simulink model "lab4"  (R2017b)
settings: Solver=FixedStepAuto  StartTime=0.0  StopTime=1  FixedStep=0.01  RelTol=1e-3
undefined symbols (not defined in the file): serial
libraries: instrumentlib x3
settings Model: Creator=Студент  LastModifiedBy=Студент

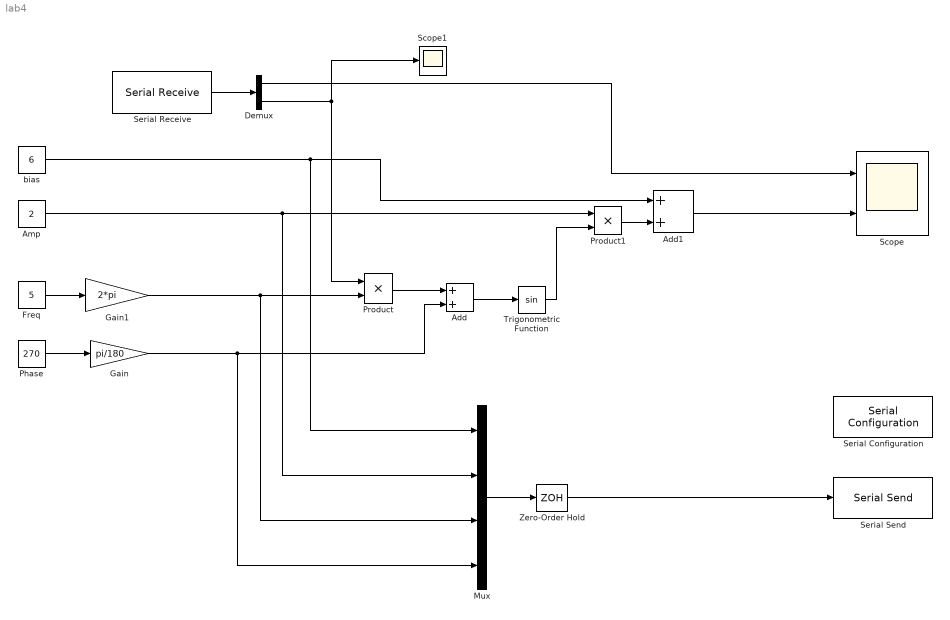
== system lab4 ==
  Add : Sum
  Add1 : Sum
  Amp : Constant  Value=2
  Demux : Demux  Outputs=2
  Freq : Constant  Value=5
  Gain : Gain  Gain=pi/180
  Gain1 : Gain  Gain=2*pi
  Mux : Mux
  Phase : Constant  Value=270
  Product : Product
  Product1 : Product
  Scope : Scope  NumInputPorts=2
  Scope1 : Scope
  Serial Configuration : instrumentlib/Serial Configuration  Priority=-200000  ComPortMenu=COM3  ComPort=COM3  ObjConstructor=serial('COM3');  BaudRate=19200  DataBits=8  Parity=none  StopBits=1  FlowControl=none  Timeout=10  ByteOrder=LittleEndian
  Serial Receive : instrumentlib/Serial Receive  ComPortMenu=COM3  ComPort=COM3  ObjConstructor=serial('COM3');  Terminator=<none>  DataSize="[1  2]"  DataType=double  EnableBlockingMode=on  ActionDataUnavailable=Output last received value  CustomValue=0  SampleTime=0.01
  Serial Send : instrumentlib/Serial Send  ComPortMenu=COM3  ComPort=COM3  ObjConstructor=serial('COM3');  Terminator=<none>  EnableBlockingMode=on
  Trigonometric Function : Trigonometry
  Zero-Order Hold : ZeroOrderHold  SampleTime=-1
  bias : Constant  Value=6  OutDataTypeStr=double
  wires:
  bias/1 -> Mux/1, Add1/1
  Amp/1 -> Mux/2, Product1/1
  Freq/1 -> Gain1/1
  Phase/1 -> Gain/1
  Product/1 -> Add/1
  Add/1 -> Trigonometric Function/1
  Trigonometric Function/1 -> Product1/2
  Product1/1 -> Add1/2
  Add1/1 -> Scope/2
  Zero-Order Hold/1 -> Serial Send/1
  Gain/1 -> Mux/4, Add/2
  Gain1/1 -> Mux/3, Product/2
  Serial Receive/1 -> Demux/1
  Demux/1 -> Scope/1
  Demux/2 -> Scope1/1, Product/1
  Mux/1 -> Zero-Order Hold/1
